simulink model "ukladRC"  (Simulink 6.6)
settings: Solver=ode113  StartTime=0.0  StopTime=6e-3
values from neighbouring files (symbols this model uses):
  C = 1e-6    (= 1e-06)    [uklad.m]    (also in uklad2.m; ukladRLC.m)
  R = 1000    [uklad.m]    (also in uklad2.m = 10; ukladRLC.m = 10)
settings Model: Creator=Student  LastModifiedBy=Student

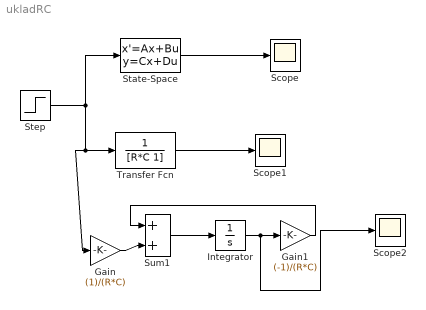
== system ukladRC ==
  Gain : Gain  Gain=(1)/(R*C)
  Gain1 : Gain  Gain=(-1)/(R*C)
  Integrator : Integrator
  Scope : Scope
      settings: TimeRange=2
  Scope1 : Scope
  Scope2 : Scope
      settings: SaveName=ScopeData2
  State-Space : StateSpace  A=(-1)/(R*C)  B=1/(R*C)  D=0
  Step : Step  Time=0  SampleTime=0
  Sum1 : Sum  Inputs=|++
  Transfer Fcn : TransferFcn  Denominator=[R*C 1]
  wires:
  Step/1 -> State-Space/1, Transfer Fcn/1, Gain/1
  Transfer Fcn/1 -> Scope1/1
  State-Space/1 -> Scope/1
  Sum1/1 -> Integrator/1
  Gain/1 -> Sum1/2
  Integrator/1 -> Gain1/1, Scope2/1
  Gain1/1 -> Sum1/1
